simulink library "ScalarProduct3D"  (R2014b)
settings: Solver=ode45  StartTime=0.0  StopTime=10.0  RelTol=1e-3
settings Model: Creator=Hp  LastModifiedBy=Hp

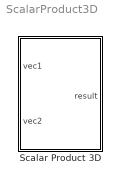
== system ScalarProduct3D ==
  Scalar Product 3D : Subsystem

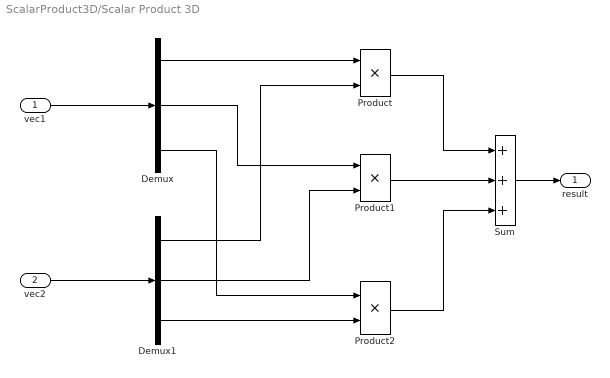
== system ScalarProduct3D/Scalar Product 3D ==
  vec1 : Inport
  vec2 : Inport  Port=2
  Demux : Demux  Outputs=3
  Demux1 : Demux  Outputs=3
  Product : Product
  Product1 : Product
  Product2 : Product
  Sum : Sum  Inputs=+++
  result : Outport
  wires:
  vec1/1 -> Demux/1
  Demux1/2 -> Product1/2
  Product1/1 -> Sum/2
  Demux/2 -> Product1/1
  Demux/1 -> Product/1
  Sum/1 -> result/1
  Product2/1 -> Sum/3
  vec2/1 -> Demux1/1
  Demux1/1 -> Product/2
  Demux1/3 -> Product2/2
  Demux/3 -> Product2/1
  Product/1 -> Sum/1
